simulink library "commeq2"  (Simulink 6.0)
settings: Solver=ode45  SolverMode=SingleTasking  StartTime=0.0  StopTime=10.0  RelTol=1e-3
undefined symbols (not defined in the file or in its folder): j, magnitude, nFwdTaps, qammod
libraries: commeqprivlib x14, dspsigops x2, simulink x2, dspsigattribs x2, dspmtrx3 x1
settings Model: Creator=ashivapr  LastModifiedBy=cvora  ExtModeAutoUpdateStatusClock=off  ProdHWDeviceType=Specified
settings DataIOCC: SignalLoggingName=logsOut
settings OptimizationCC: BooleanDataType=off
settings DebuggingCC: CheckExecutionContextPreStartOutputMsg=on  CheckExecutionContextRuntimeOutputMsg=on  SolverPrmCheckMsg=none
settings HardwareCC: ProdHWDeviceType=Specified  TargetUnknown=on
settings ModelReferenceCC: UpdateModelReferenceTargets=IfOutOfDate

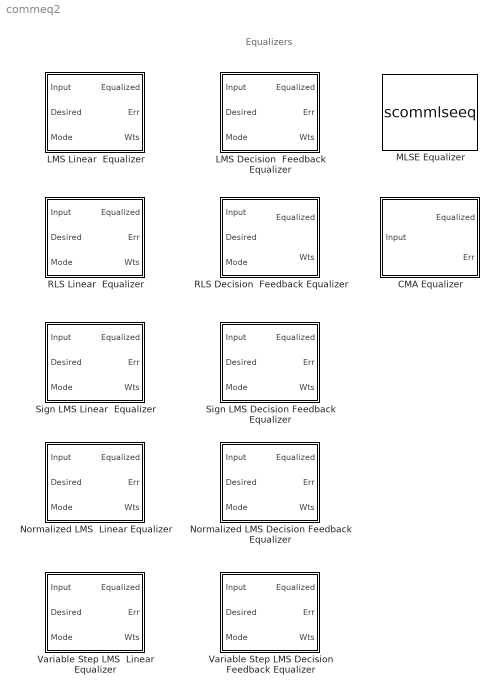
== system commeq2 ==
  note: Equalizers
  CMA Equalizer : Subsystem  PropExecContextAcrossSSBoundary=on  mask(CMA Equalizer){nTaps=4, nSamp=1, sigConst=qammod([0:15],16), stepSize=0.01, leakage=1, initWeights=[1 0 0 0], outErr=on, outWeights=off}
      mask prompts: nTaps "Number of taps:"; nSamp "Number of samples per symbol:"; sigConst "Signal constellation:"; stepSize "Step size:"; leakage "Leakage factor:"; initWeights "Initial weights:"; outErr "Output error"; outWeights "Output weights"
      mask help:
      | Equalize a linearly modulated signal through a dispersive channel using the CMA algorithm.
      |
      | The block computes filter weights with the CMA algorithm and filters the input signal. When the number of samples per symbol is 1, the filter weights are updated once for each symbol, for a symbol spaced (i.e. T-spaced) equalizer. When the number of samples per symbol is greater than one, the weights are update once every Nth sample, for a fractionally spaced (i.e. T/N-spaced) equalizer.
      |
      | The Leakage factor must be in the range 0 to 1.  A value of 1 corresponds to a conventional weight update algorithm, and a value of 0 corresponds to a memoryless update algorithm.
      mask init:
      | try
      | commblklineqmasklms
      | catch
      | 	error(lasterr)
      | end
      | commblkequpdateports
      mask Help: helpview(commbhelp)
  LMS Decision  Feedback Equalizer : Subsystem  PropExecContextAcrossSSBoundary=on  mask(LMS Decision Feedback Equalizer){nFwdTaps=6, nFdbkTaps=6, nSamp=1, sigConst=qammod([0:3],4), delay=3, stepSize=0.01, leakage=1, initWeights=0, mode=on, outErr=on, outWeights=on}
      mask prompts: nFwdTaps "Number of forward taps:"; nFdbkTaps "Number of feedback taps:"; nSamp "Number of samples per symbol:"; sigConst "Signal constellation:"; delay "Reference tap:"; stepSize "Step size:"; leakage "Leakage factor:"; initWeights "Initial weights:"; mode "Mode input port"; outErr "Output error"; outWeights "Output weights"
      mask help:
      | Equalize a linearly modulated signal through a dispersive channel using a decision feedback equalizer and the LMS algorithm.
      |
      | The block computes filter weights with the LMS algorithm and filters the input signal. The filter weights are updated once for each symbol.
      |
      | The Desired input is used for training the equalizer. It expects complex constellation points.
      |
      | The Leakage factor must be in the range 0 to 1.  A value of 1 corresponds to a conventional weight update algorithm, and a value of 0 corresponds to a memoryless update algorithm.
      |
      | If the Mode input port box is checked, the mode input toggles between training and decision directed mode. For training, the mode input must be 1, and for decision directed, the mode must be 0. For every frame in which the mode input is 1 or not present, the equalizer trains at the beginning of the frame for the length of the desired signal.
      mask init:
      | try
      | commblkdfeeqlms
      | catch
      | 	error(lasterr)
      | end
      | commblkequpdateports
      mask Help: helpview(commbhelp)
  LMS Linear  Equalizer : Subsystem  PropExecContextAcrossSSBoundary=on  mask(LMS Linear Equalizer){nTaps=4, nSamp=1, sigConst=qammod([0:15],16), delay=2, stepSize=0.01, leakage=1, initWeights=0, mode=on, outErr=on, outWeights=on}
      mask prompts: nTaps "Number of taps:"; nSamp "Number of samples per symbol:"; sigConst "Signal constellation:"; delay "Reference tap:"; stepSize "Step size:"; leakage "Leakage factor:"; initWeights "Initial weights:"; mode "Mode input port"; outErr "Output error"; outWeights "Output weights"
      mask help:
      | Equalize a linearly modulated signal through a dispersive channel using the LMS algorithm.
      |
      | The block computes filter weights with the LMS algorithm and filters the input signal. When the number of samples per symbol is 1, the filter weights are updated once for each symbol, for a symbol spaced (i.e. T-spaced) equalizer. When the number of samples per symbol is greater than one, the weights are updated once every Nth sample, for a T/N-spaced equalizer.
      |
      | The Desired input is used for training the equalizer. It expects complex constellation points.
      |
      | The Leakage factor must be in the range 0 to 1.  A value of 1 corresponds to a conventional weight update algorithm, and a value of 0 corresponds to a memoryless update algorithm.
      |
      | If the Mode input port box is checked, the mode input toggles between training and decision directed mode. For training, the mode input must be 1, and for decision directed, the mode must be 0. For every frame in which the mode input is 1 or not present, the equalizer trains at the beginning of the frame for the length of the desired signal.
      mask init:
      | try
      | commblklineqmasklms
      | catch
      | 	error(lasterr)
      | end
      | commblkequpdateports
      mask Help: helpview(commbhelp)
  MLSE Equalizer : S-Function  FunctionName=scommlseeq  Parameters=specchan, real(chancoeff), imag(chancoeff), real(cplxconstpts), imag(cplxconstpts), tbdepth, opmode, enpreamble, preamble, enpostamble, postamble, numsamp, reset  SFunctionModules=viterbi_acs_tbdec  mask(MLSE Equalizer){specchan=Dialog, chancoeff=[1 0.7 0.5 0.3]', constpts=[1+j -1+j -1-j 1-j], tbdepth=21, opmode=Continuous with reset option, enpreamble=off, preamble=[0 3 2 1], enpostamble=off, postamble=[0 2 3 1], numsamp=1, reset=off}
      mask prompts: specchan "Specify channel via:"; chancoeff "Channel coefficients:"; constpts "Signal constellation:"; tbdepth "Traceback depth:"; opmode "Operation mode:"; enpreamble "Input contains preamble"; preamble "Expected preamble:"; enpostamble "Input contains postamble"; postamble "Expected postamble:"; numsamp "Samples per input symbol:"; reset "Enable the reset input port"
      mask help:
      | Equalize a linearly modulated signal through a dispersive channel using the Viterbi algorithm.
      |
      | The block estimates the transmitted sequence from the received signal and the channel estimates, and then outputs complex constellation points at the symbol rate.
      mask init:
      | [e, s, cplxconstpts] = commblkmlseeq(gcb,'init');
      | if ~isempty(e.msg)
      | 	error(e.msg); 
      | end
      mask Help: helpview(commbhelp)
      mask StyleString: popup(Input port|Dialog),edit,edit,edit,popup(Continuous with reset option|Reset every frame),checkbox,edit,checkbox,edit,edit,checkbox
      mask CallbackString: commblkmlseeq(gcb,'cbSpecchan');||||commblkmlseeq(gcb,'cbOpmode');|commblkmlseeq(gcb,'cbEnpreamble');||commblkmlseeq(gcb,'cbEnpostamble');|||
      mask Display:
      | plot(-10,-10,110,110,s.draw.x,s.draw.y);
      | disp('\n\nMLSE Equalizer');
      | port_label('input',s.ports.i1,s.ports.i1s);
      | port_label('input',s.ports.i2,s.ports.i2s);
      | port_label('input',s.ports.i3,s.ports.i3s);
      | port_label('output',s.ports.o1,s.ports.o1s);
  Normalized LMS Decision Feedback Equalizer : Subsystem  PropExecContextAcrossSSBoundary=on  mask(Normalized LMS Decision Feedback Equalizer){nFwdTaps=6, nFdbkTaps=6, nSamp=1, sigConst=qammod([0:3],4), delay=3, stepSize=0.01, leakage=1, bias=0, initWeights=0, mode=on, outErr=on, outWeights=on}
      mask prompts: nFwdTaps "Number of forward taps:"; nFdbkTaps "Number of feedback taps:"; nSamp "Number of samples per symbol:"; sigConst "Signal constellation:"; delay "Reference tap:"; stepSize "Step size:"; leakage "Leakage factor:"; initWeights "Initial weights:"; mode "Mode input port"; outErr "Output error"; outWeights "Output weights"
      mask help:
      | Equalize a linearly modulated signal through a dispersive channel using a decision feedback equalizer and the normalized LMS algorithm.
      |
      | The block computes filter weights with the normalized LMS algorithm and filters the input signal. When the number of samples per symbol is 1, the filter weights are updated once for each symbol, for a symbol spaced (i.e. T-spaced) equalizer. When the number of samples per symbol is greater than one, the weights are updated once every Nth sample, for a T/N-spaced equalizer.
      |
      | The Desired input is used for training the equalizer. It expects complex constellation points.
      |
      | The Leakage factor must be in the range 0 to 1.  A value of 1 corresponds to a conventional weight update algorithm, and a value of 0 corresponds to a memoryless update algorithm.
      |
      | If the Mode Input box is checked, the mode input toggles between training and decision directed mode. For training, the mode input must be 1, for decision directed, the mode should be 0. The equalizer will train for the length of the Desired signal. If the mode input is not present, the equalizer will train at the beginning of every frame for the length of the Desired signal.
      mask init:
      | try
      | commblkdfeeqlms
      | catch
      | 	error(lasterr)
      | end
      | if(~isnumeric(bias) || ~isscalar(bias) || bias < 0 )
      | 	error('Bias must be a numeric scalar greater than 0.');
      | end
      | commblkequpdateports
      mask Help: helpview(commbhelp)
  Normalized LMS  Linear Equalizer : Subsystem  PropExecContextAcrossSSBoundary=on  mask(Normalized LMS Linear Equalizer){nTaps=4, nSamp=1, sigConst=qammod([0:15],16), delay=2, stepSize=0.01, leakage=1, bias=1, initWeights=0, mode=on, outErr=on, outWeights=on}
      mask prompts: nTaps "Number of taps:"; nSamp "Number of samples per symbol:"; sigConst "Signal constellation:"; delay "Reference tap:"; stepSize "Step size:"; leakage "Leakage factor:"; initWeights "Initial weights:"; mode "Mode input port"; outErr "Output error"; outWeights "Output weights"
      mask help:
      | Equalize a linearly modulated signal through a dispersive channel using the normalized LMS algorithm.
      |
      | The block computes filter weights with the normalized LMS algorithm and filters the input signal. When the number of samples per symbol is 1, the filter weights are updated once for each symbol, for a symbol spaced (i.e. T-spaced) equalizer. When the number of samples per symbol is greater than one, the weights are updated once every Nth sample, for a T/N-spaced equalizer.
      |
      | The Desired input is used for training the equalizer. It expects complex constellation points.
      |
      | The Leakage factor must be in the range 0 to 1.  A value of 1 corresponds to a conventional weight update algorithm, and a value of 0 corresponds to a memoryless update algorithm.
      |
      | If the Mode Input box is checked, the mode input toggles between training and decision directed mode. For training, the mode input must be 1, for decision directed, the mode should be 0. For every frame in which the mode input is 1 or not present, the equalizer trains at the beginning of the frame for the length of the desired signal.
      mask init:
      | try
      | commblklineqmasklms
      | catch
      | 	error(lasterr)
      | end
      | 
      | if(~isnumeric(bias) || ~isscalar(bias) || bias < 0 )
      | 	error('Bias must be a numeric scalar greater than 0.');
      | end
      | commblkequpdateports
      mask Help: helpview(commbhelp)
  RLS Decision  Feedback Equalizer : Subsystem  PropExecContextAcrossSSBoundary=on  mask(RLS Decision Feedback equalizer){nFwdTaps=2, nFdbkTaps=2, nSamp=1, sigConst=qammod([0:15],16), delay=1, lambda=.99, invCorr=.1*eye(4), initWeights=0, mode=on, outErr=off, outWeights=on}
      mask prompts: nFwdTaps "Number of forward taps:"; nFdbkTaps "Number of feedback taps:"; nSamp "Number of samples per symbol:"; sigConst "Signal constellation:"; delay "Reference tap:"; lambda "Forgetting factor:"; invCorr "Inverse correlation matrix"; initWeights "Initial weights:"; mode "Mode input port"; outErr "Output error"; outWeights "Output weights"
      mask help:
      | Equalize a linearly modulated signal through a dispersive channel using a decision feedback equalizer and the RLS algorithm.
      |
      | The block computes filter weights with the RLS algorithm and filters the input signal. When the number of samples per symbol is 1, the filter weights are updated once for each symbol, for a symbol spaced equalizer. When the number of samples per symbol is greater than one, the weights are update once every Nth sample, for a fractionally spaced equalizer.
      |
      | The Desired input is used for training the equalizer. It expects complex constellation points.
      |
      | If the Mode input port box is checked, the mode input toggles between training and decision directed mode. For training, the mode input must be 1, and for decision directed, the mode must be 0. For every frame in which the mode input is 1 or not present, the equalizer trains at the beginning of the frame for the length of the desired signal.
      mask init:
      | try
      | commblkdfeeqrls
      | catch
      | 	error(lasterr)
      | end
      | commblkequpdateports
      mask Help: helpview(commbhelp)
  RLS Linear  Equalizer : Subsystem  PropExecContextAcrossSSBoundary=on  mask(RLS Linear Equalizer){nTaps=4, nSamp=1, sigConst=qammod([0:15],16), delay=2, lambda=.99, invCorr=.1*eye(4), initWeights=0, mode=on, outErr=on, outWeights=on}
      mask prompts: nTaps "Number of taps:"; nSamp "Number of samples per symbol:"; sigConst "Signal constellation:"; delay "Reference tap:"; lambda "Forgetting factor:"; invCorr "Inverse correlation matrix"; initWeights "Initial weights:"; mode "Mode input port"; outErr "Output error"; outWeights "Output weights"
      mask help:
      | Equalize a linearly modulated signal through a dispersive channel using the RLS algorithm.
      |
      | The block computes filter weights with the RLS algorithm and filters the input signal. When the number of samples per symbol is 1, the filter weights are updated once for each symbol, for a symbol spaced (i.e. T-spaced) equalizer. When the number of samples per symbol is greater than one, the weights are updated once every Nth sample, for a fractionally spaced (i.e. T/N-spaced) equalizer.
      |
      | The Desired input is used for training the equalizer. It expects complex constellation points.
      |
      | If the Mode input port box is checked, the mode input toggles between training and decision directed mode. For training, the mode input must be 1, and for decision directed, the mode must be 0. For every frame in which the mode input is 1 or not present, the equalizer trains at the beginning of the frame for the length of the desired signal.
      mask init:
      | try
      | commblklineqmaskrls
      | catch
      | 	error(lasterr)
      | end
      | commblkequpdateports
      mask Help: helpview(commbhelp)
  Sign LMS Decision Feedback Equalizer : Subsystem  PropExecContextAcrossSSBoundary=on  mask(Sign LMS Decision Feedback Equalizer){alg=Sign LMS, nFwdTaps=4, nFdbkTaps=4, nSamp=1, sigConst=qammod([0:15],16), delay=2, stepSize=0.01, leakage=1, initWeights=0, mode=on, outErr=on, outWeights=on}
      mask prompts: alg "Update algorithm"; nFwdTaps "Number of forward taps:"; nFdbkTaps "Number of feedback taps:"; nSamp "Number of samples per symbol:"; sigConst "Signal constellation:"; delay "Reference tap:"; stepSize "Step size:"; leakage "Leakage factor:"; initWeights "Initial weights:"; mode "Mode input port"; outErr "Output error"; outWeights "Output weights"
      mask help:
      | Equalize a linearly modulated signal through a dispersive channel using a decision feedback equalizer and the signed LMS algorithm.
      |
      | The block computes filter weights with the signed LMS algorithm and filters the input signal. When the number of samples per symbol is 1, the filter weights are updated once for each symbol, for a symbol spaced (i.e. T-spaced) equalizer. When the number of samples per symbol is greater than one, the weights are updated once every Nth sample, for a T/N-spaced equalizer.
      |
      | The Desired input is used for training the equalizer. It expects complex constellation points.
      |
      | The Leakage factor must be in the range 0 to 1.  A value of 1 corresponds to a conventional weight update algorithm, and a value of 0 corresponds to a memoryless update algorithm.
      |
      | If the Mode Input box is checked, the mode input toggles between training and decision directed mode. For training, the mode input must be 1, for decision directed, the mode should be 0. For every frame in which the mode input is 1 or not present, the equalizer trains at the beginning of the frame for the length of the desired signal.
      mask init:
      | try
      | commblkdfeeqlms
      | catch
      | 	error(lasterr)
      | end
      | commblkequpdateports
      mask Help: helpview(commbhelp)
      mask StyleString: popup(Sign LMS|Sign Regressor LMS|Sign Sign LMS),edit,edit,edit,edit,edit,edit,edit,edit,checkbox,checkbox,checkbox
      mask CallbackString: commblkeqsignlms|||||||||||
  Sign LMS Linear  Equalizer : Subsystem  PropExecContextAcrossSSBoundary=on  mask(Sign LMS Linear Equalizer){alg=Sign LMS, nTaps=4, nSamp=1, sigConst=qammod([0:15],16), delay=2, stepSize=0.01, leakage=1, initWeights=0, mode=on, outErr=on, outWeights=on}
      mask prompts: alg "Update algorithm"; nTaps "Number of taps:"; nSamp "Number of samples per symbol:"; sigConst "Signal constellation:"; delay "Reference tap:"; stepSize "Step size:"; leakage "Leakage factor:"; initWeights "Initial weights:"; mode "Mode input port"; outErr "Output error"; outWeights "Output weights"
      mask help:
      | Equalize a linearly modulated signal through a dispersive channel using the signed LMS algorithm.
      |
      | The block computes filter weights with the signed LMS algorithm and filters the input signal. When the number of samples per symbol is 1, the filter weights are updated once for each symbol, for a symbol spaced (i.e. T-spaced) equalizer. When the number of samples per symbol is greater than one, the weights are updated once every Nth sample, for a T/N-spaced equalizer.
      |
      | The Desired input is used for training the equalizer. It expects complex constellation points.
      |
      | The Leakage factor must be in the range 0 to 1.  A value of 1 corresponds to a conventional weight update algorithm, and a value of 0 corresponds to a memoryless update algorithm.
      |
      | If the Mode Input box is checked, the mode input toggles between training and decision directed mode. For training, the mode input must be 1, for decision directed, the mode should be 0. For every frame in which the mode input is 1 or not present, the equalizer trains at the beginning of the frame for the length of the desired signal.
      mask init:
      | try
      | commblklineqmasklms
      | catch
      | 	error(lasterr)
      | end
      | commblkequpdateports
      mask Help: helpview(commbhelp)
      mask StyleString: popup(Sign LMS|Sign Regressor LMS|Sign Sign LMS),edit,edit,edit,edit,edit,edit,edit,checkbox,checkbox,checkbox
      mask CallbackString: commblkeqsignlms||||||||||
  Variable Step LMS Decision Feedback Equalizer : Subsystem  PropExecContextAcrossSSBoundary=on  mask(Variable Step LMS Decision Feedback Equalizer){nFwdTaps=6, nFdbkTaps=6, nSamp=1, sigConst=qammod([0:3],4), delay=3, initMu=.01, incMu=.001, minMu=.001, maxMu=.1, leakage=1, initWeights=0, mode=on, outErr=on, outWeights=on}
      mask prompts: nFwdTaps "Number of forward taps:"; nFdbkTaps "Number of feedback taps:"; nSamp "Number of samples per symbol:"; sigConst "Signal constellation:"; delay "Reference tap:"; initMu "Initial step size:"; incMu "Increment step size:"; minMu "Minumum step size:"; maxMu "Maximum step size:"; leakage "Leakage factor:"; initWeights "Initial weights:"; mode "Mode input port"; outErr "Output error"; outWeights "Output weights"
      mask help:
      | Equalize a linearly modulated signal through a dispersive channel using a decision feedback equalizer and the variable step LMS algorithm.
      |
      | The block computes filter weights with the variable step LMS algorithm and filters the input signal. When the number of samples per symbol is 1, the filter weights are updated once for each symbol, for a symbol spaced (i.e. T-spaced) equalizer. When the number of samples per symbol is greater than one, the weights are updated once every Nth sample, for a T/N-spaced equalizer.
      |
      | The Desired input is used for training the equalizer. It expects complex constellation points.
      |
      | The Leakage factor must be in the range 0 to 1.  A value of 1 corresponds to a conventional weight update algorithm, and a value of 0 corresponds to a memoryless update algorithm.
      |
      | If the Mode Input box is checked, the mode input toggles between training and decision directed mode. For training, the mode input must be 1, for decision directed, the mode should be 0. The equalizer will train for the length of the Desired signal. If the mode input is not present, the equalizer will train at the beginning of every frame for the length of the Desired signal.
      mask init:
      | try
      | 	commblklineqmaskvarlms
      | catch
      | 	error(laster)
      | end
      | 
      | try
      | 	commblkdfeeqlms
      | catch
      | 	error(lasterr)
      | end
      | 
      | commblkequpdateports
      mask Help: helpview(commbhelp)
  Variable Step LMS  Linear Equalizer : Subsystem  PropExecContextAcrossSSBoundary=on  mask(Variable Step LMS Linear Equalizer){nTaps=4, nSamp=1, sigConst=qammod([0:15],16), delay=2, initMu=.01, incMu=.01, minMu=.001, maxMu=.1, leakage=1, initWeights=0, mode=on, outErr=on, outWeights=on}
      mask prompts: nTaps "Number of taps:"; nSamp "Number of samples per symbol:"; sigConst "Signal constellation:"; delay "Reference tap:"; initMu "Initial step size:"; incMu "Increment step size:"; minMu "Minimum step size:"; maxMu "Maximum step size:"; leakage "Leakage factor:"; initWeights "Initial weights:"; mode "Mode input port"; outErr "Output error"; outWeights "Output weights"
      mask help:
      | Equalize a linearly modulated signal through a dispersive channel using the variable step LMS algorithm.
      |
      | The block computes filter weights with the variable step LMS algorithm and filters the input signal. When the number of samples per symbol is 1, the filter weights are updated once for each symbol, for a symbol spaced (i.e. T-spaced) equalizer. When the number of samples per symbol is greater than one, the weights are updated once every Nth sample, for a T/N-spaced equalizer.
      |
      | The Desired input is used for training the equalizer. It expects complex constellation points.
      |
      | The Leakage factor must be in the range 0 to 1.  A value of 1 corresponds to a conventional weight update algorithm, and a value of 0 corresponds to a memoryless update algorithm.
      |
      | If the Mode Input box is checked, the mode input toggles between training and decision directed mode. For training, the mode input must be 1, for decision directed, the mode should be 0. For every frame in which the mode input is 1 or not present, the equalizer trains at the beginning of the frame for the length of the desired signal.
      mask init:
      | try
      | 	commblklineqmaskvarlms
      | catch
      | 	error(lasterr)
      | end
      | 
      | try
      | 	commblklineqmasklms
      | catch
      | 	error(lasterr)
      | end
      | 
      | commblkequpdateports
      mask Help: helpview(commbhelp)

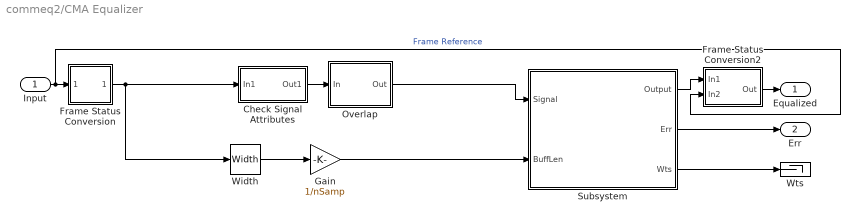
== system commeq2/CMA Equalizer ==
  Input : Inport  LatchInput=off
  Check Signal Attributes : Subsystem  PropExecContextAcrossSSBoundary=on  mask(Check Signal Attributes){SigAttribCheckMethod=Does not match attributes exactly, Complexity=Complex, Frame=Ignore, DimsCheckMethod=Is not..., Dimensions=Full matrix (2-D), DatatypeCheckMethod=Ignore, DatatypeGeneral=Boolean, DtypeFloatSpecific=Any floating-point, DtypeFixedSpecific=Any fixed-point, DtypeIntSpecific=Any integer, SampleMode=Ignore}
      mask prompts: SigAttribCheckMethod "Error when input:"; Frame "Frame status:"; DimsCheckMethod "Dimensionality:"; DatatypeCheckMethod "Data type:"; DatatypeGeneral "General data type:"; DtypeFloatSpecific "Specific floating-point:"; DtypeFixedSpecific "Specific fixed-point:"; DtypeIntSpecific "Specific integer:"; SampleMode "Sample mode:"
      mask help: Generate an error when the input signal does or does not match selected attributes exactly.
      mask Help: web(dspbhelp);
      mask StyleString: popup(Does not match attributes exactly|Matches attributes exactly),popup(Ignore|Real|Complex),popup(Ignore|Frame-based|Sample-based),popup(Ignore|Is...|Is not...),popup(1-D|2-D|Scalar (1-D or 2-D)|Vector (1-D or 2-D)|Vector (1-D or 2-D) or scalar|Row vector (2-D)|Row vector (2-D) or scalar|Column vector (2-D)|Column vector (2-D) or scalar|Full matrix (2-D)|Square matrix (2-D)),popup(Ignore|Is...|Is not...),popup(Boolean|Floating-point|Fixed-point|Integer),popup(Any floating-point|Double precision|Single precision),popup(Any fixed-point|Signed fixed-point|Unsigned fixed-point),popup(Any integer|Signed integer|Unsigned integer|int8|int16|int32|uint8|uint16|uint32),popup(Ignore|Discrete|Continuous)
      mask CallbackString: |||dspblkchksigattrbs||dspblkchksigattrbs|dspblkchksigattrbs|||dspblkchksigattrbs|
      mask Display: disp('Check Signal\n Attributes');
  Frame Status Conversion : Subsystem  PropExecContextAcrossSSBoundary=on  mask(Frame Status Conversion){growRefPort=off, outframe=Frame-based}
      mask prompts: growRefPort "Inherit output frame status from Ref input port"; outframe "Output signal:"
      mask help: Specify the frame status of the output signal.
      mask init:
      | [p, str] = dspblkfrmconv('init');
      mask Help: web(dspbhelp);
      mask StyleString: checkbox,popup(Frame-based|Sample-based)
      mask CallbackString: dspblkfrmconv|
      mask Display:
      | port_label(p.in1,   p.i1,  p.i1s);
      | port_label(p.in2,   p.i2,  p.i2s);
      | port_label(p.out, p.o1, p.o1s);
      | disp(str)
  Frame Status Conversion2 : Subsystem  PropExecContextAcrossSSBoundary=on  mask(Frame Status Conversion){growRefPort=on, outframe=Frame-based}
      mask prompts: growRefPort "Inherit output frame status from Ref input port"; outframe "Output signal:"
      mask help: Specify the frame status of the output signal.
      mask init:
      | [p, str] = dspblkfrmconv('init');
      mask Help: web(dspbhelp);
      mask StyleString: checkbox,popup(Frame-based|Sample-based)
      mask CallbackString: dspblkfrmconv|
      mask Display:
      | port_label(p.in1,   p.i1,  p.i1s);
      | port_label(p.in2,   p.i2,  p.i2s);
      | port_label(p.out, p.o1, p.o1s);
      | disp(str)
  Gain : Gain  Gain=1/nSamp  SaturateOnIntegerOverflow=on
  Overlap : Subsystem  PropExecContextAcrossSSBoundary=on
  Subsystem : Subsystem  PropExecContextAcrossSSBoundary=on
  Width : Width
  Wts : Terminator
  Equalized : Outport
  Err : Outport  Port=2
  wires:
  Check Signal Attributes/1(Out1) -> Overlap/1(In)
  Width/1 -> Gain/1
  Input/1 -> Frame Status Conversion2/2(In2), Frame Status Conversion/1(In1)  "Frame Reference"
  Overlap/1(Out) -> Subsystem/1(Signal)
  Gain/1 -> Subsystem/2(BuffLen)
  Subsystem/2(Err) -> Err/1
  Subsystem/3(Wts) -> Wts/1
  Subsystem/1(Output) -> Frame Status Conversion2/1(In1)
  Frame Status Conversion2/1(Out) -> Equalized/1
  Frame Status Conversion/1(Out) -> Check Signal Attributes/1(In1), Width/1

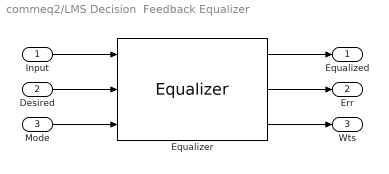
== system commeq2/LMS Decision  Feedback Equalizer ==
  Input : Inport  LatchInput=off
  Desired : Inport  Port=2  LatchInput=off
  Mode : Inport  Port=3  LatchInput=off
  "Equalizer " : commeqprivlib/Equalizer   eqType=DFE  alg=LMS
  Equalized : Outport
  Err : Outport  Port=2
  Wts : Outport  Port=3
  wires:
  Input/1 -> "Equalizer "/1
  Desired/1 -> "Equalizer "/2
  Mode/1 -> "Equalizer "/3
  "Equalizer "/1 -> Equalized/1
  "Equalizer "/2 -> Err/1
  "Equalizer "/3 -> Wts/1

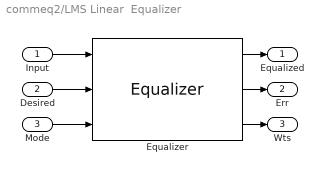
== system commeq2/LMS Linear  Equalizer ==
  Input : Inport  LatchInput=off
  Desired : Inport  Port=2  LatchInput=off
  Mode : Inport  Port=3  LatchInput=off
  "Equalizer " : commeqprivlib/Equalizer   eqType=Linear  alg=LMS
  Equalized : Outport
  Err : Outport  Port=2
  Wts : Outport  Port=3
  wires:
  Input/1 -> "Equalizer "/1
  Desired/1 -> "Equalizer "/2
  Mode/1 -> "Equalizer "/3
  "Equalizer "/1 -> Equalized/1
  "Equalizer "/2 -> Err/1
  "Equalizer "/3 -> Wts/1

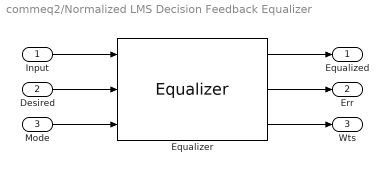
== system commeq2/Normalized LMS Decision Feedback Equalizer ==
  Input : Inport  LatchInput=off
  Desired : Inport  Port=2  LatchInput=off
  Mode : Inport  Port=3  LatchInput=off
  "Equalizer " : commeqprivlib/Equalizer   eqType=DFE  alg=Normalized LMS
  Equalized : Outport
  Err : Outport  Port=2
  Wts : Outport  Port=3
  wires:
  "Equalizer "/3 -> Wts/1
  "Equalizer "/2 -> Err/1
  "Equalizer "/1 -> Equalized/1
  Mode/1 -> "Equalizer "/3
  Desired/1 -> "Equalizer "/2
  Input/1 -> "Equalizer "/1

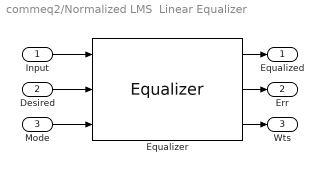
== system commeq2/Normalized LMS  Linear Equalizer ==
  Input : Inport  LatchInput=off
  Desired : Inport  Port=2  LatchInput=off
  Mode : Inport  Port=3  LatchInput=off
  "Equalizer " : commeqprivlib/Equalizer   eqType=Linear  alg=Normalized LMS
  Equalized : Outport
  Err : Outport  Port=2
  Wts : Outport  Port=3
  wires:
  "Equalizer "/3 -> Wts/1
  "Equalizer "/2 -> Err/1
  "Equalizer "/1 -> Equalized/1
  Mode/1 -> "Equalizer "/3
  Desired/1 -> "Equalizer "/2
  Input/1 -> "Equalizer "/1

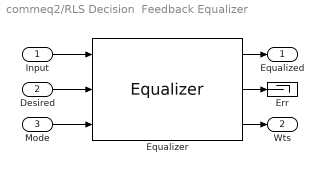
== system commeq2/RLS Decision  Feedback Equalizer ==
  Input : Inport  LatchInput=off
  Desired : Inport  Port=2  LatchInput=off
  Mode : Inport  Port=3  LatchInput=off
  "Equalizer " : commeqprivlib/Equalizer   eqType=DFE  alg=RLS
  Err : Terminator
  Equalized : Outport
  Wts : Outport  Port=2
  wires:
  Input/1 -> "Equalizer "/1
  Desired/1 -> "Equalizer "/2
  Mode/1 -> "Equalizer "/3
  "Equalizer "/1 -> Equalized/1
  "Equalizer "/2 -> Err/1
  "Equalizer "/3 -> Wts/1

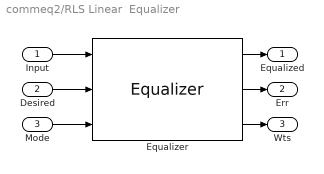
== system commeq2/RLS Linear  Equalizer ==
  Input : Inport  LatchInput=off
  Desired : Inport  Port=2  LatchInput=off
  Mode : Inport  Port=3  LatchInput=off
  "Equalizer " : commeqprivlib/Equalizer   eqType=Linear  alg=RLS
  Equalized : Outport
  Err : Outport  Port=2
  Wts : Outport  Port=3
  wires:
  "Equalizer "/3 -> Wts/1
  "Equalizer "/2 -> Err/1
  "Equalizer "/1 -> Equalized/1
  Mode/1 -> "Equalizer "/3
  Desired/1 -> "Equalizer "/2
  Input/1 -> "Equalizer "/1

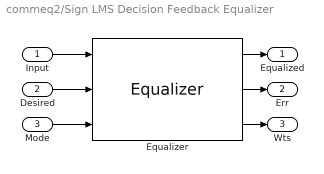
== system commeq2/Sign LMS Decision Feedback Equalizer ==
  Input : Inport  LatchInput=off
  Desired : Inport  Port=2  LatchInput=off
  Mode : Inport  Port=3  LatchInput=off
  "Equalizer " : commeqprivlib/Equalizer   eqType=DFE  alg=Sign LMS
  Equalized : Outport
  Err : Outport  Port=2
  Wts : Outport  Port=3
  wires:
  Input/1 -> "Equalizer "/1
  Desired/1 -> "Equalizer "/2
  Mode/1 -> "Equalizer "/3
  "Equalizer "/1 -> Equalized/1
  "Equalizer "/2 -> Err/1
  "Equalizer "/3 -> Wts/1

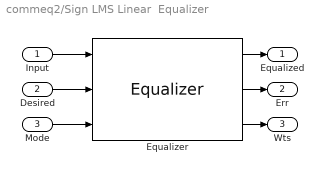
== system commeq2/Sign LMS Linear  Equalizer ==
  Input : Inport  LatchInput=off
  Desired : Inport  Port=2  LatchInput=off
  Mode : Inport  Port=3  LatchInput=off
  "Equalizer " : commeqprivlib/Equalizer   eqType=Linear  alg=Sign LMS
  Equalized : Outport
  Err : Outport  Port=2
  Wts : Outport  Port=3
  wires:
  "Equalizer "/3 -> Wts/1
  "Equalizer "/2 -> Err/1
  "Equalizer "/1 -> Equalized/1
  Mode/1 -> "Equalizer "/3
  Desired/1 -> "Equalizer "/2
  Input/1 -> "Equalizer "/1

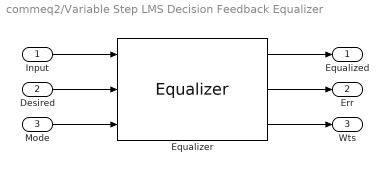
== system commeq2/Variable Step LMS Decision Feedback Equalizer ==
  Input : Inport  LatchInput=off
  Desired : Inport  Port=2  LatchInput=off
  Mode : Inport  Port=3  LatchInput=off
  "Equalizer " : commeqprivlib/Equalizer   eqType=DFE  alg=Variable Step LMS
  Equalized : Outport
  Err : Outport  Port=2
  Wts : Outport  Port=3
  wires:
  Input/1 -> "Equalizer "/1
  Desired/1 -> "Equalizer "/2
  Mode/1 -> "Equalizer "/3
  "Equalizer "/1 -> Equalized/1
  "Equalizer "/2 -> Err/1
  "Equalizer "/3 -> Wts/1

== system commeq2/Variable Step LMS  Linear Equalizer ==
  Input : Inport  LatchInput=off
  Desired : Inport  Port=2  LatchInput=off
  Mode : Inport  Port=3  LatchInput=off
  "Equalizer " : commeqprivlib/Equalizer   eqType=Linear  alg=Variable Step LMS
  Equalized : Outport
  Err : Outport  Port=2
  Wts : Outport  Port=3
  wires:
  Input/1 -> "Equalizer "/1
  Desired/1 -> "Equalizer "/2
  Mode/1 -> "Equalizer "/3
  "Equalizer "/1 -> Equalized/1
  "Equalizer "/2 -> Err/1
  "Equalizer "/3 -> Wts/1

== system commeq2/CMA Equalizer/Check Signal Attributes ==
  In1 : Inport  LatchInput=off
  Check Signal Attributes : S-Function  FunctionName=sdspsigattrib  Parameters=SigAttribCheckMethod,Complexity,Frame,DimsCheckMethod,Dimensions,DatatypeCheckMethod,DatatypeGeneral,DtypeFloatSpecific,DtypeFixedSpecific,DtypeIntSpecific,SampleMode
  Out1 : Outport
  wires:
  In1/1 -> Check Signal Attributes/1, Out1/1

== system commeq2/CMA Equalizer/Frame Status Conversion ==
  In1 : Inport  LatchInput=off
  Frame Status : FrameConversion
  Out : Outport
  wires:
  Frame Status/1 -> Out/1
  In1/1 -> Frame Status/1

== system commeq2/CMA Equalizer/Frame Status Conversion2 ==
  In1 : Inport  LatchInput=off
  In2 : Inport  Port=2  LatchInput=off
  Inherit : S-Function  FunctionName=sdspfrmconv  Parameters=growRefPort,outframe
  Out : Outport
  wires:
  In1/1 -> Inherit/1
  Inherit/1 -> Out/1
  In2/1 -> Inherit/2

== system commeq2/CMA Equalizer/Overlap ==
  note: This subsystem appends nTaps samples
      | to the input signal. The purpose of this is to remember
      | the previous nTaps sampes, as they are needed to
      | compute the current weights.
  In : Inport  LatchInput=off
  Delay2 : dspsigops/Delay  Orientation=left  dly_unit=Samples  delay=nFwdTaps  ic_detail=off  dif_ic_for_ch=off  dif_ic_for_dly=off  ic=0  reset_popup=None
  Matrix Concatenation : simulink/Math Operations/Matrix Concatenation  numInports=2  catMethod=Vertical
  Signal Specification : simulink/Signal Attributes/Signal Specification  Orientation=down  D=[nFwdTaps 1]  Ts=-1  DataType=auto  OutDataType=sfix(16)  OutScaling=2^0
      settings: SignalType=auto  SamplingMode=auto
  Submatrix : dspmtrx3/Submatrix  Orientation=up  RowSpan=Range of rows  RowStartMode=Offset from last  RowStartIndex=nFwdTaps-1  RowEndMode=Last  RowEndIndex=1  ColSpan=Range of columns  ColStartMode=First  ColStartIndex=1  ColEndMode=Last  ColEndIndex=1
  Out : Outport
  wires:
  Signal Specification/1 -> Matrix Concatenation/1
  Matrix Concatenation/1 -> Submatrix/1, Out/1
  Delay2/1 -> Signal Specification/1
  Submatrix/1 -> Delay2/1
  In/1 -> Matrix Concatenation/2

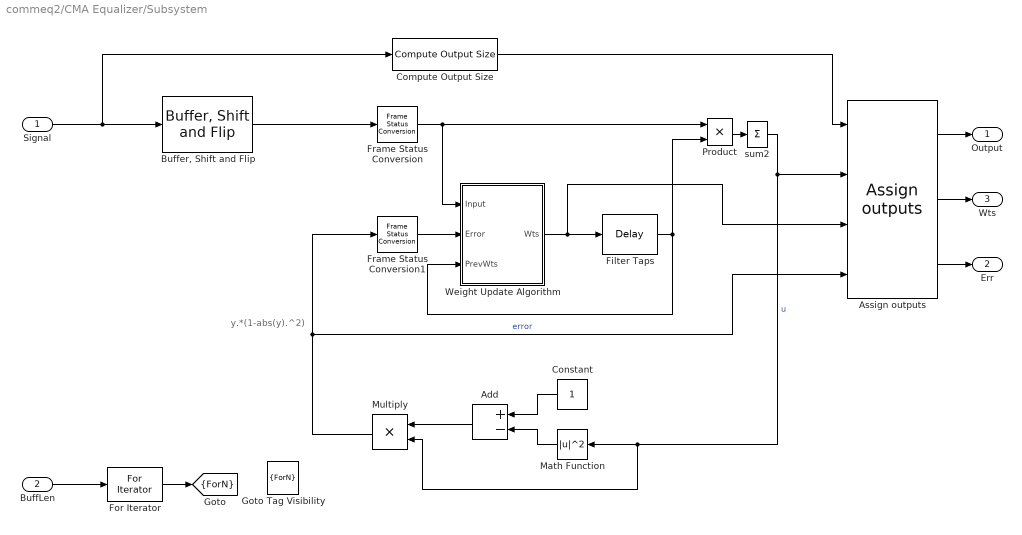
== system commeq2/CMA Equalizer/Subsystem ==
  note: y.*(1-abs(y).^2)
  Signal : Inport  LatchInput=off
  BuffLen : Inport  Port=2  LatchInput=off
  Add : Sum  Orientation=left  Inputs=+-  OutScaling=2^-10
  Assign outputs : commeqprivlib/Assign outputs
  "Buffer, Shift and Flip" : commeqprivlib/Buffer, Shift and Flip
  Compute Output Size : commeqprivlib/Compute Output Size
  Constant : Constant  Orientation=left
  Filter Taps : dspsigops/Delay  dly_unit=Samples  delay=1  ic_detail=on  dif_ic_for_ch=on  dif_ic_for_dly=off  ic=initWeights  reset_popup=None
  For Iterator : ForIterator  IterationSource=external  IterationLimit=4  IndexMode=Zero-based  IterationVariableDataType=double
  Frame Status Conversion : dspsigattribs/Frame Status Conversion  growRefPort=off  outframe=Sample-based
  Frame Status Conversion1 : dspsigattribs/Frame Status Conversion  growRefPort=off  outframe=Sample-based
  Goto Tag Visibility : GotoTagVisibility  GotoTag=ForN
  Math Function : Math  Orientation=left  Operator=magnitude^2  SaturateOnIntegerOverflow=on
  Multiply : Product  Orientation=left  Inputs=**  OutScaling=2^-10
  Product : Product  SaturateOnIntegerOverflow=on
  Weight Update Algorithm : Subsystem  BlockChoice=LMS  PropExecContextAcrossSSBoundary=on
      settings: AttributesFormatString=%<BlockChoice>  TemplateBlock=commeqprivlib/Weight Update Algorithm  MemberBlocks=Complex Sign LMS,LMS,Normalized LMS,RLS,Sign LMS,Sign Regressor LMS,Sign Sign LMS,Variable Step LMS
  sum2 : Sum  Inputs=+  SaturateOnIntegerOverflow=on  InputSameDT=on
  Output : Outport
  Err : Outport  Port=2
  Wts : Outport  Port=3
  tag scope: ForN=scoped
  wires:
  Frame Status Conversion1/1 -> Weight Update Algorithm/2(Error)
  Frame Status Conversion/1 -> Weight Update Algorithm/1(Input), Product/1
  "Buffer, Shift and Flip"/1 -> Frame Status Conversion/1
  Assign outputs/3 -> Err/1
  Product/1 -> sum2/1
  Weight Update Algorithm/1(Wts) -> Assign outputs/3, Filter Taps/1
  Filter Taps/1 -> Weight Update Algorithm/3(PrevWts), Product/2
  sum2/1 -> Assign outputs/2, Math Function/1, Multiply/2  "u"
  Assign outputs/2 -> Wts/1
  Signal/1 -> "Buffer, Shift and Flip"/1, Compute Output Size/1
  Compute Output Size/1 -> Assign outputs/1
  Assign outputs/1 -> Output/1
  BuffLen/1 -> For Iterator/1
  For Iterator/1 -> [ForN]
  Constant/1 -> Add/1
  Math Function/1 -> Add/2
  Add/1 -> Multiply/1
  Multiply/1 -> Frame Status Conversion1/1, Assign outputs/4  "error"

== system commeq2/CMA Equalizer/Subsystem/Weight Update Algorithm ==
  Input : Inport  LatchInput=off
  Error : Inport  Port=2  LatchInput=off
  PrevWts : Inport  Port=3  LatchInput=off
  LMS : commeqprivlib/LMS
  Wts : Outport
  wires:
  Input/1 -> LMS/1
  Error/1 -> LMS/2
  PrevWts/1 -> LMS/3
  LMS/1 -> Wts/1
